simulink model "ODU_zad1"  (Simulink 6.3)
settings: Solver=ode45  StartTime=0.0  StopTime=5  RelTol=1e-3
settings Model: LastModifiedBy=Ms1

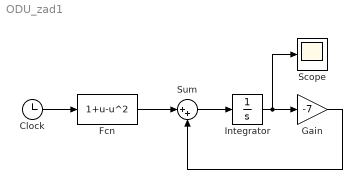
== system ODU_zad1 ==
  Clock : Clock
      settings: Decimation=10
  Fcn : Fcn  Expr=1+u-u^2
  Gain : Gain  Gain=-7  SaturateOnIntegerOverflow=on
  Integrator : Integrator  InitialCondition=-4
  Scope : Scope
  Sum : Sum  Inputs=|++  SaturateOnIntegerOverflow=on  InputSameDT=on
  wires:
  Integrator/1 -> Gain/1, Scope/1
  Gain/1 -> Sum/2
  Sum/1 -> Integrator/1
  Clock/1 -> Fcn/1
  Fcn/1 -> Sum/1
